simulink model "PSO_ZVD"  (R2021a)
settings: Solver=VariableStepAuto  StartTime=0.0  StopTime=20  RelTol=1e-3
InitFcn:
  | ml=2;
  | 
  | mc=0.5;
  | M2=0.5;
  | 
  | mt=5;
  | g=9.81;
  | l_ref=0.1;
  | l_ini=1;
  | l=l_ini;
  | x_ref=1;
  | n1=5;n2=1;
  | 
  | %ADRC' s parameter caculation
  | %b0 = (ml+mc)/(mc*ml +mc*mt+ml*mt); %Hieu
  | b0=(ml+mc)/(mt*mc+2*ml*mc+mt*ml+ml^2+mc^2); %Enhanced-coupling
  | k_ESO = 100;
  | T_set  = 6;
  | 
  | s_cl = -5.85/T_set;
  | Kp   = s_cl^2;
  | Kd   = -2*s_cl;
  | 
  | s_ESO = k_ESO*s_cl;
  | l1        = -3*s_ESO;
  | l2        = 3*( s_ESO)^2;
  | l3        = -(s_ESO)^3;
  | 
  | %b1 = (mt+mc)/(mc*ml +mc*mt+ml*mt);
  | b1=1/(ml+mc);
  | k_ESO1 =100;
  | T_set1  = 3;
  | s_cl1 = -5.85/T_set1;
  | Kp1   = s_cl1^2;
  | Kd1   = -2*s_cl1;
  | 
  | s_ESO1 = k_ESO1*s_cl1;
  | l11        = -3*s_ESO1;
  | l21        = 3*( s_ESO1)^2;
  | l31        = -(s_ESO1)^3;
  | 
  | 
  | L1=l_ini;
  | %L2=0.5;
  | L2=0.1;
  | m1=2;
  | m2=mc;
  | m=5;
  | %Bo input shaping
  | alpha = (1/L1 + 1/L2)*(m1+M2)/m1;
  | beta = (((m1+M2)/m1)^2)*((1/L1 + 1/L2)^2) - 4*(m1+M2)/(m1*L1*L2);
  | w1 = sqrt(g*(alpha - sqrt(beta))/2);
  | w2 = sqrt(g*(alpha + sqrt(beta))/2);
  | damping_ratio = 0;
  | wd1 = w1*sqrt(1-damping_ratio^2);
  | wd2 = w2*sqrt(1-damping_ratio^2);
  | k = exp(damping_ratio*pi/sqrt(1-damping_ratio^2));
  | 
  | %ZVD1
  | t1_ZVD_1=pi/wd1;
  | t2_ZVD_1=2*pi/wd1;
  | 
  | %ETM4_1
  | m_etm4_1 = 0.1;
  | I_etm4_1 = (1+m_etm4_1)*k*k/(k^2 + (1+m_etm4_1)*(k^(4/3)+k^(2/3)) + m_etm4_1);
  | A1_etm4_1 = I_etm4_1/(1+m_etm4_1);
  | A2_etm4_1 = I_etm4_1/(k^(2/3));
  | A3_etm4_1 = I_etm4_1/(k^(4/3));
  | A4_etm4_1 = m_etm4_1*I_etm4_1/((1+m_etm4_1)*(k^2));
  | t1_etm4_1 = (2*pi/3)/wd1;
  | t2_etm4_1 = (4*pi/3)/wd1;
  | t3_etm4_1 = 2*pi/wd1;
  | 
  | %ZVD1
  | t1_ZVD_2=pi/wd2;
  | t2_ZVD_2=2*pi/wd2;
  | 
  | %ETM4_2
  | m_etm4_2 = 0.1;
  | I_etm4_2 = (1+m_etm4_2)*k*k/(k^2 + (1+m_etm4_2)*(k^(4/3)+k^(2/3)) + m_etm4_2);
  | A1_etm4_2 = I_etm4_2/(1+m_etm4_2);
  | A2_etm4_2 = I_etm4_2/(k^(2/3));
  | A3_etm4_2 = I_etm4_2/(k^(4/3));
  | A4_etm4_2 = m_etm4_2*I_etm4_2/((1+m_etm4_2)*(k^2));
  | t1_etm4_2 = (2*pi/3)/wd2;
  | t2_etm4_2 = (4*pi/3)/wd2;
  | t3_etm4_2 = 2*pi/wd2;
values from neighbouring files (symbols this model uses):
  particle = repmat(empty_particle, nPop, 1)    [PSO16_12.m]    (also in PSO_ZVD.m)
undefined symbols (not defined in the file or in its folder): i, li, xi
libraries: neural x101, simulink_extras x13, simulink x3
(part 1 of 34)
settings Model: Creator=Dao Hieu  LastModifiedBy=Admin

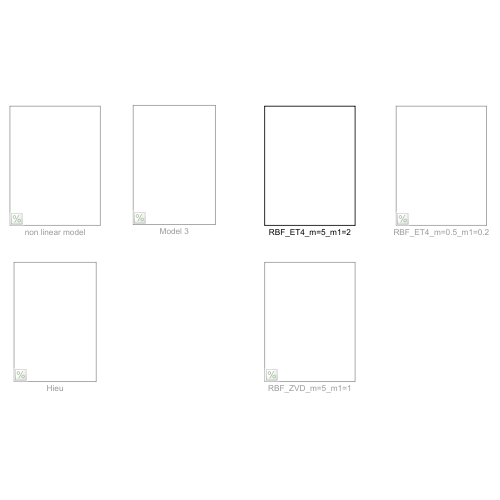
[thumbnail: Simulink's stored preview of the top-level diagram]
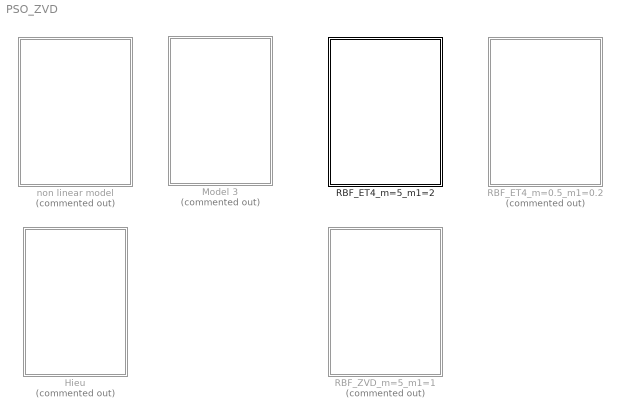
== system PSO_ZVD ==
  Hieu : Subsystem  Commented=on
  Model 3 : Subsystem  Commented=on
  RBF_ET4_m=0.5_m1=0.2 : Subsystem  Commented=on
  RBF_ET4_m=5_m1=2 : Subsystem
  RBF_ZVD_m=5_m1=1 : Subsystem  Commented=on
  non linear model : Subsystem  Commented=on

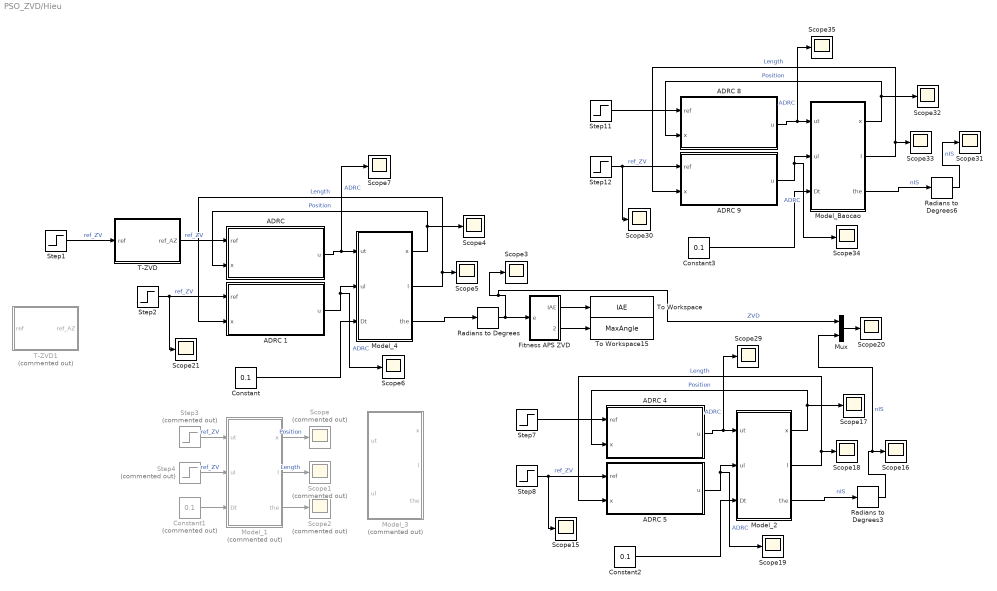
== system PSO_ZVD/Hieu ==
  "ADRC " : Subsystem
  ADRC 1 : Subsystem
  ADRC 4 : Subsystem
  ADRC 5 : Subsystem
  ADRC 8 : Subsystem
  ADRC 9 : Subsystem
  Constant : Constant  Value=0.1
  Constant1 : Constant  Commented=on  Value=0.1
  Constant2 : Constant  Value=0.1
  Constant3 : Constant  Value=0.1
  Fitness APS ZVD : Subsystem
  Model_1 : Subsystem  Commented=on
  Model_2 : Subsystem
  Model_3 : Subsystem  Commented=on
  Model_4 : Subsystem
  Model_Baocao : Subsystem
  Mux : Mux  Inputs=2
  Radians to Degrees : simulink_extras/Transformations/Radians to Degrees
  Radians to Degrees3 : simulink_extras/Transformations/Radians to Degrees
  Radians to Degrees6 : simulink_extras/Transformations/Radians to Degrees
  Scope : Scope  Commented=on
  Scope1 : Scope  Commented=on
  Scope{3..7,15..21,29..35} (19 alike) : Scope
  Scope2 : Scope  Commented=on
  Step1 : Step  SampleTime=0
  Step11 : Step  SampleTime=0
  Step12 : Step  Before=l_ini  After=l_ref  SampleTime=0
  Step2 : Step  Before=l_ini  After=l_ref  SampleTime=0
  Step3 : Step  Commented=on  SampleTime=0
  Step4 : Step  Commented=on  Before=l  After=l  SampleTime=0
  Step7 : Step  SampleTime=0
  Step8 : Step  Before=l_ini  After=l_ref  SampleTime=0
  T-ZVD : Subsystem
  T-ZVD1 : Subsystem  Commented=on
  To Workspace : ToWorkspace  VariableName=IAE  SampleTime=-1
  To Workspace15 : ToWorkspace  VariableName=MaxAngle  SampleTime=-1
  wires:
  Model_1/1(x) -> Scope/1  "Position"
  Fitness APS ZVD/1(IAE) -> To Workspace/1
  Model_4/2(l) -> Scope5/1, ADRC 1/2(x)  "Length"
  Model_Baocao/2(l) -> Scope33/1, ADRC 9/2(x)  "Length"
  Constant1/1 -> Model_1/3(Dt)
  Model_4/1(x) -> Scope4/1, "ADRC "/2(x)  "Position"
  Step8/1 -> ADRC 5/1(ref), Scope15/1  "ref_ZV"
  ADRC 1/1(u) -> Scope6/1, Model_4/2(ul)  "ADRC"
  Model_1/3(the) -> Scope2/1
  Step2/1 -> Scope21/1, ADRC 1/1(ref)  "ref_ZV"
  T-ZVD/1(ref_AZ) -> "ADRC "/1(ref)  "ref_ZV"
  Constant/1 -> Model_4/3(Dt)
  Step7/1 -> ADRC 4/1(ref)
  Step1/1 -> T-ZVD/1(ref)  "ref_ZV"
  Fitness APS ZVD/2(MAx) -> To Workspace15/1
  "ADRC "/1(u) -> Scope7/1, Model_4/1(ut)  "ADRC"
  ADRC 8/1(u) -> Scope35/1, Model_Baocao/1(ut)  "ADRC"
  Radians to Degrees/1 -> Mux/1, Scope3/1, Fitness APS ZVD/1(e)  "ZVD"
  ADRC 4/1(u) -> Scope29/1, Model_2/1(ut)  "ADRC"
  Step12/1 -> Scope30/1, ADRC 9/1(ref)  "ref_ZV"
  Constant2/1 -> Model_2/3(Dt)
  Model_4/3(the) -> Radians to Degrees/1
  Model_Baocao/1(x) -> Scope32/1, ADRC 8/2(x)  "Position"
  Step3/1 -> Model_1/1(ut)  "ref_ZV"
  Model_1/2(l) -> Scope1/1  "Length"
  ADRC 5/1(u) -> Scope19/1, Model_2/2(ul)  "ADRC"
  Constant3/1 -> Model_Baocao/3(Dt)
  Radians to Degrees3/1 -> Mux/2, Scope16/1  "nIS"
  Step11/1 -> ADRC 8/1(ref)
  ADRC 9/1(u) -> Scope34/1, Model_Baocao/2(ul)  "ADRC"
  Model_2/2(l) -> ADRC 5/2(x), Scope18/1  "Length"
  Radians to Degrees6/1 -> Scope31/1  "nIS"
  Mux/1 -> Scope20/1
  Step4/1 -> Model_1/2(ul)  "ref_ZV"
  Model_2/1(x) -> ADRC 4/2(x), Scope17/1  "Position"
  Model_2/3(the) -> Radians to Degrees3/1  "nIS"
  Model_Baocao/3(the) -> Radians to Degrees6/1  "nIS"

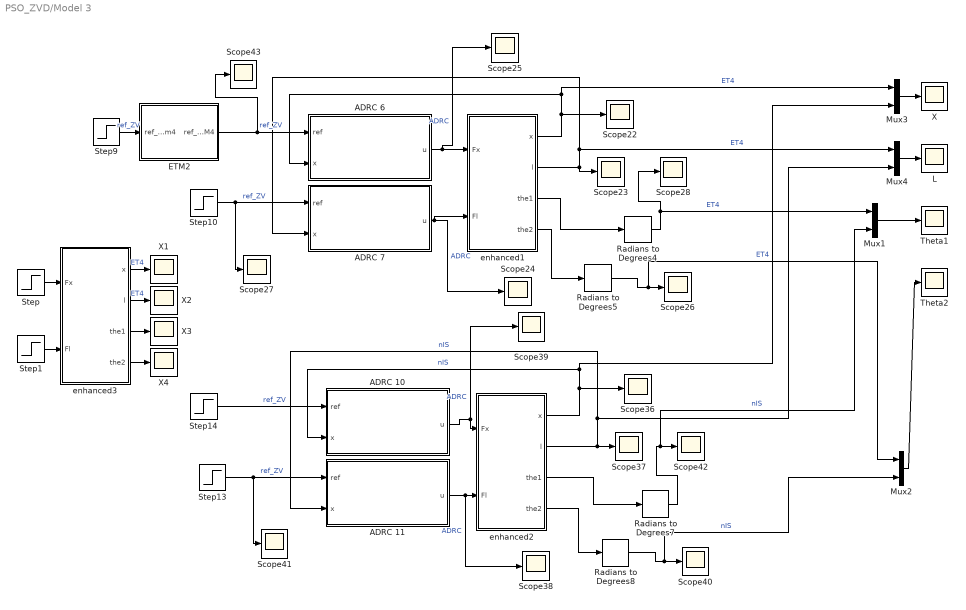
== system PSO_ZVD/Model 3 ==
  ADRC 10 : Subsystem
  ADRC 11 : Subsystem
  ADRC 6 : Subsystem
  ADRC 7 : Subsystem
  ETM2 : Subsystem
  L : Scope
  Mux{1..4} (4 alike) : Mux  Inputs=2
  Radians to Degrees{4..5,7..8} (4 alike) : simulink_extras/Transformations/Radians to Degrees
  Scope{22..28,36..43} (15 alike) : Scope
  Step : Step  Time=0  After=0  SampleTime=0
  Step1 : Step  Time=0  SampleTime=0
  Step10 : Step  Time=0  Before=l_ini  After=l_ref  SampleTime=0
  Step13 : Step  Time=0  Before=l_ini  After=l_ref  SampleTime=0
  Step14 : Step  Time=0  After=x_ref  SampleTime=0
  Step9 : Step  Time=0  After=x_ref  SampleTime=0
  Theta1 : Scope
  Theta2 : Scope
  X{,1..4} (5 alike) : Scope
  enhanced1 : Subsystem
  enhanced2 : Subsystem
  enhanced3 : Subsystem
  wires:
  Radians to Degrees4/1 -> Mux1/1, Scope28/1  "ET4"
  enhanced1/3(the1) -> Radians to Degrees4/1
  ADRC 6/1(u) -> enhanced1/1(Fx), Scope25/1  "ADRC"
  Radians to Degrees7/1 -> Mux1/2, Scope42/1  "nIS"
  Step13/1 -> Scope41/1, ADRC 11/1(ref)  "ref_ZV"
  Radians to Degrees5/1 -> Mux2/1, Scope26/1  "ET4"
  ADRC 11/1(u) -> enhanced2/2(Fl), Scope38/1  "ADRC"
  ADRC 7/1(u) -> enhanced1/2(Fl), Scope24/1  "ADRC"
  ETM2/1(ref_ETM4) -> Scope43/1, ADRC 6/1(ref)  "ref_ZV"
  enhanced2/1(x) -> Scope36/1, Mux3/2, ADRC 10/2(x)  "nIS"
  Step9/1 -> ETM2/1(ref_ETm4)  "ref_ZV"
  Mux1/1 -> Theta1/1
  Step14/1 -> ADRC 10/1(ref)  "ref_ZV"
  Mux2/1 -> Theta2/1
  enhanced1/4(the2) -> Radians to Degrees5/1
  enhanced2/3(the1) -> Radians to Degrees7/1
  Step10/1 -> Scope27/1, ADRC 7/1(ref)  "ref_ZV"
  ADRC 10/1(u) -> enhanced2/1(Fx), Scope39/1  "ADRC"
  Radians to Degrees8/1 -> Mux2/2, Scope40/1  "nIS"
  enhanced2/4(the2) -> Radians to Degrees8/1
  Mux3/1 -> X/1
  enhanced1/1(x) -> Scope22/1, Mux3/1, ADRC 6/2(x)  "ET4"
  enhanced2/2(l) -> Scope37/1, Mux4/2, ADRC 11/2(x)  "nIS"
  enhanced1/2(l) -> Scope23/1, ADRC 7/2(x), Mux4/1  "ET4"
  Mux4/1 -> L/1
  enhanced3/1(x) -> X1/1  "ET4"
  enhanced3/2(l) -> X2/1  "ET4"
  enhanced3/3(the1) -> X3/1
  enhanced3/4(the2) -> X4/1
  Step/1 -> enhanced3/1(Fx)
  Step1/1 -> enhanced3/2(Fl)

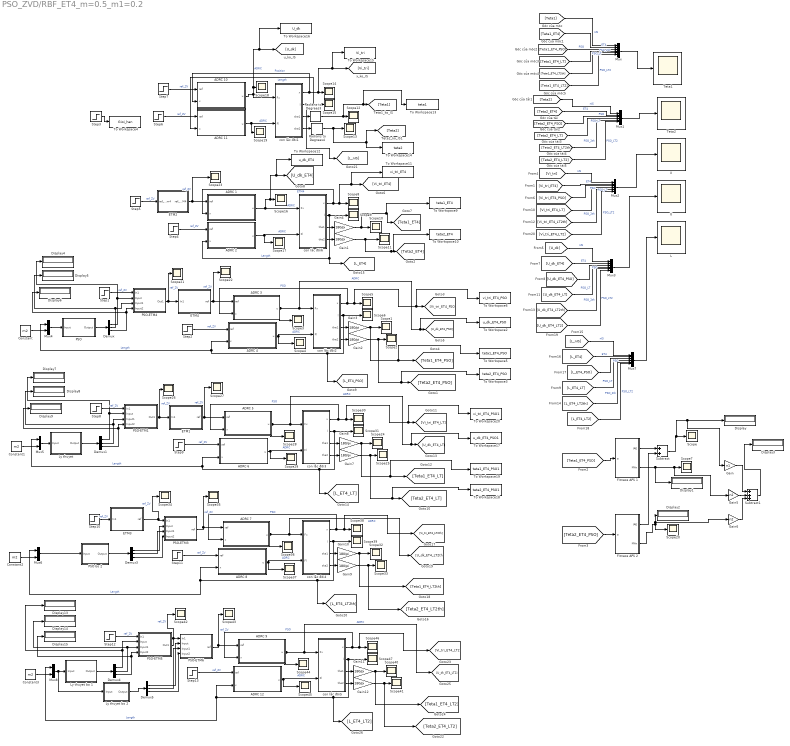
== system PSO_ZVD/RBF_ET4_m=0.5_m1=0.2 ==
  ADRC 1 : Subsystem
  ADRC 10 : Subsystem
  ADRC 11 : Subsystem
  ADRC 12 : Subsystem
  ADRC 2 : Subsystem
  ADRC 3 : Subsystem
  ADRC 4 : Subsystem
  ADRC 5 : Subsystem
  ADRC 6 : Subsystem
  ADRC 7 : Subsystem
  ADRC 8 : Subsystem
  ADRC 9 : Subsystem
  Constant{,1..3} (4 alike) : Constant  Value=m2
  Demux{,1,3..5} (5 alike) : Demux  Outputs=3
  Display{,1..9,13..15} (13 alike) : Display
  ETM1 : Subsystem
  ETM2 : Subsystem
  ETM3 : Subsystem
  ETM4 : Subsystem
  Fitness APS 1 : Subsystem
  Fitness APS 2 : Subsystem
  Gain : Gain  Gain=n1
  Gain{1..4,7..12} (10 alike) : Gain  Gain=180/pi
  Gain5 : Gain  Gain=n2
  Gain6 : Gain  Gain=n2
  L : Scope
  Ly thuyet : Subsystem
      mask help: Radial Basis Network
      mask Display: e = 0.06;c1 = [120 150 230]/255;c2 = ([120 150 230]+0)/383;c3 = ([120 150 230]+128)/383;patch([0 1 1 0],[0 0 1 1],c1);patch([0 1 1 1-e 1-e 0+e],[0 0 1 1-e 0+e 0+e],c2);patch([0 0 1 1-e 0+e 0+e],[0 1 1 1-e 1-e 0+e],c3);plot([0 1 1 0 0],[0 0 1 1 0]);fprintf('NNET');port_label('input',1,' Input');port_label('output',1,'Output ');
  Ly thuyet bo 1 : Subsystem
      mask help: Radial Basis Network
      mask Display: e = 0.06;c1 = [120 150 230]/255;c2 = ([120 150 230]+0)/383;c3 = ([120 150 230]+128)/383;patch([0 1 1 0],[0 0 1 1],c1);patch([0 1 1 1-e 1-e 0+e],[0 0 1 1-e 0+e 0+e],c2);patch([0 0 1 1-e 0+e 0+e],[0 1 1 1-e 1-e 0+e],c3);plot([0 1 1 0 0],[0 0 1 1 0]);fprintf('NNET');port_label('input',1,' Input');port_label('output',1,'Output ');
  Ly thuyet bo 2 : Subsystem
      mask help: Radial Basis Network
      mask Display: e = 0.06;c1 = [120 150 230]/255;c2 = ([120 150 230]+0)/383;c3 = ([120 150 230]+128)/383;patch([0 1 1 0],[0 0 1 1],c1);patch([0 1 1 1-e 1-e 0+e],[0 0 1 1-e 0+e 0+e],c2);patch([0 0 1 1-e 0+e 0+e],[0 1 1 1-e 1-e 0+e],c3);plot([0 1 1 0 0],[0 0 1 1 0]);fprintf('NNET');port_label('input',1,' Input');port_label('output',1,'Output ');
  Mux{,1..3,7} (5 alike) : Mux  Inputs=6
  Mux{4..6,8} (4 alike) : Mux  Inputs=2
  PSO : Subsystem
      mask help: Radial Basis Network
      mask Display: e = 0.06;c1 = [120 150 230]/255;c2 = ([120 150 230]+0)/383;c3 = ([120 150 230]+128)/383;patch([0 1 1 0],[0 0 1 1],c1);patch([0 1 1 1-e 1-e 0+e],[0 0 1 1-e 0+e 0+e],c2);patch([0 0 1 1-e 0+e 0+e],[0 1 1 1-e 1-e 0+e],c3);plot([0 1 1 0 0],[0 0 1 1 0]);fprintf('NNET');port_label('input',1,' Input');port_label('output',1,'Output ');
  PSO bo 2 : Subsystem
      mask help: Radial Basis Network
      mask Display: e = 0.06;c1 = [120 150 230]/255;c2 = ([120 150 230]+0)/383;c3 = ([120 150 230]+128)/383;patch([0 1 1 0],[0 0 1 1],c1);patch([0 1 1 1-e 1-e 0+e],[0 0 1 1-e 0+e 0+e],c2);patch([0 0 1 1-e 0+e 0+e],[0 1 1 1-e 1-e 0+e],c3);plot([0 1 1 0 0],[0 0 1 1 0]);fprintf('NNET');port_label('input',1,' Input');port_label('output',1,'Output ');
  PSO-ETM1 : Subsystem
  PSO-ETM3 : Subsystem
  PSO-ETM4 : Subsystem
  PSO-ETM5 : Subsystem
  PSO-ETM6 : Subsystem
  Radians to Degrees3 : simulink_extras/Transformations/Radians to Degrees
  Radians to Degrees4 : simulink_extras/Transformations/Radians to Degrees
  Scope{,1..47} (48 alike) : Scope
  Step{1,5,7..8,10,12} (6 alike) : Step  Time=0  After=x_ref  SampleTime=0
  Step{2,4,6,9,11,13} (6 alike) : Step  Time=0  Before=l_ini  After=l_ref  SampleTime=0
  Step3 : Step  Time=0  After=10  SampleTime=0
  Subtract : Sum
  Subtract1 : Sum  Inputs=+++
  Teta1 : Scope
  Teta2 : Scope
  To Workspace10 : ToWorkspace  VariableName=teta2_ET4  SaveFormat=Timeseries  SampleTime=-1
  To Workspace11 : ToWorkspace  VariableName=vi_tri_ET4  SaveFormat=Timeseries  SampleTime=-1
  To Workspace12 : ToWorkspace  VariableName=u_dk_ET4  SaveFormat=Timeseries  SampleTime=-1
  To Workspace13 : ToWorkspace  VariableName=teta1  SaveFormat=Timeseries  SampleTime=-1
  To Workspace14 : ToWorkspace  VariableName=teta2  SaveFormat=Timeseries  SampleTime=-1
  To Workspace15 : ToWorkspace  VariableName=Vi_tri  SaveFormat=Timeseries  SampleTime=-1
  To Workspace16 : ToWorkspace  VariableName=U_dk  SaveFormat=Timeseries  SampleTime=-1
  To Workspace17 : ToWorkspace  VariableName=u_dk_ET4_PSO1  SaveFormat=Timeseries  SampleTime=-1
  To Workspace18 : ToWorkspace  VariableName=teta2_ET4_PSO1  SaveFormat=Timeseries  SampleTime=-1
  To Workspace19 : ToWorkspace  VariableName=teta1_ET4_PSO1  SaveFormat=Timeseries  SampleTime=-1
  To Workspace2 : ToWorkspace  VariableName=u_dk_ET4_PSO  SaveFormat=Timeseries  SampleTime=-1
  To Workspace20 : ToWorkspace  VariableName=vi_tri_ET4_PSO1  SaveFormat=Timeseries  SampleTime=-1
  To Workspace3 : ToWorkspace  VariableName=teta2_ET4_PSO  SaveFormat=Timeseries  SampleTime=-1
  To Workspace4 : ToWorkspace  VariableName=Gioi_han  SaveFormat=Timeseries  SampleTime=-1
  To Workspace5 : ToWorkspace  VariableName=teta1_ET4_PSO  SaveFormat=Timeseries  SampleTime=-1
  To Workspace6 : ToWorkspace  VariableName=vi_tri_ET4_PSO  SaveFormat=Timeseries  SampleTime=-1
  To Workspace9 : ToWorkspace  VariableName=teta1_ET4  SaveFormat=Timeseries  SampleTime=-1
  U : Scope
  X : Scope
  con lắc đôi1 : Subsystem
  con lắc đôi2 : Subsystem
  con lắc đôi3 : Subsystem
  con lắc đôi4 : Subsystem
  con lắc đôi5 : Subsystem
  con lắc đôi6 : Subsystem
  wires:
  ADRC 2/1(u) -> con lắc đôi6/2(Fl), Scope17/1  "ADRC"
  ADRC 11/1(u) -> con lắc đôi1/2(Fl), Scope19/1  "ADRC"
  ADRC 1/1(u) -> con lắc đôi6/1(Fx), To Workspace12/1, [U_dk_ET4], Scope16/1  "ADRC"
  con lắc đôi6/1(x) -> ADRC 1/2(x), To Workspace11/1, [Vi_tri_ET4], Scope8/1  "ETM4"
  con lắc đôi1/3(the1) -> Radians to Degrees3/1
  con lắc đôi6/2(l) -> [L_ET4], ADRC 2/2(x), Scope9/1  "Length"
  con lắc đôi1/1(x) -> ADRC 10/2(x), To Workspace15/1, [Vi_tri], Scope14/1  "Position"
  Step6/1 -> ADRC 11/1(ref)  "ref_ZV"
  Step4/1 -> ADRC 2/1(ref)  "ref_ZV"
  con lắc đôi1/2(l) -> Scope15/1, ADRC 11/2(x), [L_nIS]  "Length"
  Step7/1 -> ADRC 10/1(ref)  "ref_ZV"
  Gain4/1 -> To Workspace9/1, [Teta1_ET4], Scope10/1
  ETM2/1(ref_ETM4) -> ADRC 1/1(ref), Scope23/1  "ref_ZV"
  Step5/1 -> ETM2/1(ref_ETm4)  "ref_ZV"
  ADRC 10/1(u) -> con lắc đôi1/1(Fx), To Workspace16/1, [U_dk], Scope18/1  "ADRC"
  Radians to Degrees3/1 -> To Workspace13/1, [Teta1], Scope12/1
  con lắc đôi1/4(the2) -> Radians to Degrees4/1
  con lắc đôi6/3(the1) -> Gain4/1
  Gain1/1 -> To Workspace10/1, [Teta2_ET4], Scope11/1
  con lắc đôi6/4(the2) -> Gain1/1
  Radians to Degrees4/1 -> [Teta2], To Workspace14/1, Scope13/1
  ADRC 4/1(u) -> con lắc đôi2/2(Fl), Scope4/1  "ADRC"
  con lắc đôi2/4(the2) -> Gain2/1
  Step1/1 -> PSO-ETM4/1(In1)  "ref_ZV"
  ADRC 3/1(u) -> Scope3/1, con lắc đôi2/1(Fx), To Workspace2/1, [U_dk_ET4_PSO]  "ADRC"
  con lắc đôi2/1(x) -> ADRC 3/2(x), To Workspace6/1, [Vi_tri_ET4_PSO], Scope5/1  "PSO"
  con lắc đôi2/2(l) -> Scope6/1, [L_ET4_PSO], ADRC 4/2(x), Mux4/1  "Length"
  Gain3/1 -> [Teta1_ET4_PSO], To Workspace5/1, Scope1/1
  Step2/1 -> ADRC 4/1(ref)  "ref_ZV"
  con lắc đôi2/3(the1) -> Gain3/1
  PSO-ETM4/1(Out1) -> Scope21/1, ETM4/1(In1)  "ref_ZV"
  [Teta2] -> Mux1/1  "nIS"
  Subtract/1 -> Gain/1, Display/1, Scope/1
  [U_dk] -> Mux3/1  "nIS"
  [U_dk_ET4] -> Mux3/2  "ET4"
  [Teta2_ET4_PSO] -> Fitness APS 2/1(e)
  [Teta1_ET4_PSO] -> Fitness APS 1/1(e)
  [Vi_tri] -> Mux2/1  "nIS"
  [Teta2_ET4] -> Mux1/2  "ET4"
  [Vi_tri_ET4] -> Mux2/2  "ET4"
  [Teta1] -> Mux/1  "nIS"
  Gain5/1 -> Subtract1/2
  Fitness APS 2/2(MAx) -> Gain6/1, Display2/1, Scope20/1
  Mux2/1 -> X/1
  Gain6/1 -> Subtract1/3
  Mux/1 -> Teta1/1
  Mux1/1 -> Teta2/1
  Mux3/1 -> U/1
  Gain/1 -> Subtract1/1
  [Teta1_ET4] -> Mux/2  "ET4"
  Fitness APS 2/1(IAE) -> Subtract/2
  Subtract1/1 -> Display3/1
  Fitness APS 1/1(IAE) -> Subtract/1
  Fitness APS 1/2(MAx) -> Display1/1, Gain5/1, Scope7/1
  Step3/1 -> To Workspace4/1
  Gain2/1 -> [Teta2_ET4_PSO], To Workspace3/1, Scope2/1
  [Teta2_ET4_PSO] -> Mux1/3  "PSO"
  [Vi_tri_ET4_PSO] -> Mux2/3  "PSO"
  [Teta1_ET4_PSO] -> Mux/3  "PSO"
  [U_dk_ET4_PSO] -> Mux3/3  "PSO"
  Constant/1 -> Mux4/2
  Mux4/1 -> PSO/1(Input)
  Demux/1 -> PSO-ETM4/2(Input), Display4/1
  Demux/2 -> Display5/1, PSO-ETM4/3(Input1)
  Demux/3 -> Display6/1, PSO-ETM4/4(Input2)
  ETM4/1(ref) -> ADRC 3/1(ref), Scope22/1  "ref_ZV"
  PSO/1(Output) -> Demux/1
  Demux1/1 -> PSO-ETM1/2(Input), Display7/1
  Mux5/1 -> Ly thuyet/1(Input)
  Constant1/1 -> Mux5/2
  con lắc đôi3/1(x) -> ADRC 5/2(x), To Workspace20/1, [Vi_tri_ET4_LT], Scope30/1  "PSO"
  Gain7/1 -> [Teta2_ET4_LT], To Workspace18/1, Scope25/1
  con lắc đôi3/3(the1) -> Gain8/1
  Step9/1 -> ADRC 6/1(ref)  "ref_ZV"
  ETM1/1(ref) -> ADRC 5/1(ref), Scope27/1  "ref_ZV"
  PSO-ETM1/1(Out1) -> Scope26/1, ETM1/1(In1)  "ref_ZV"
  ADRC 5/1(u) -> Scope28/1, con lắc đôi3/1(Fx), To Workspace17/1, [U_dk_ET4_LT]  "ADRC"
  Demux1/2 -> Display8/1, PSO-ETM1/3(Input1)
  Demux1/3 -> Display9/1, PSO-ETM1/4(Input2)
  ADRC 6/1(u) -> con lắc đôi3/2(Fl), Scope29/1  "ADRC"
  con lắc đôi3/2(l) -> Scope31/1, [L_ET4_LT], ADRC 6/2(x), Mux5/1  "Length"
  Ly thuyet/1(Output) -> Demux1/1
  Gain8/1 -> [Teta1_ET4_LT], To Workspace19/1, Scope24/1
  con lắc đôi3/4(the2) -> Gain7/1
  Step8/1 -> PSO-ETM1/1(In1)  "ref_ZV"
  [Teta1_ET4_LT] -> Mux/4  "PSO_LT"
  [Teta2_ET4_LT] -> Mux1/4  "PSO_LT"
  [Vi_tri_ET4_LT] -> Mux2/4  "PSO_LT"
  [U_dk_ET4_LT] -> Mux3/4  "PSO_LT"
  PSO-ETM3/1(ref) -> ADRC 7/1(ref), Scope35/1  "ref_ZV"
  Step11/1 -> ADRC 8/1(ref)  "ref_ZV"
  Demux3/1 -> PSO-ETM3/2(Input)
  Demux3/2 -> PSO-ETM3/3(Input1)
  ETM3/1(ref) -> PSO-ETM3/1(In1), Scope34/1  "ref_ZV"
  con lắc đôi4/2(l) -> Scope39/1, [L_ET4_LT2th], ADRC 8/2(x), Mux6/1  "Length"
  Gain10/1 -> [Teta1_ET4_LT2th], Scope32/1
  ADRC 8/1(u) -> con lắc đôi4/2(Fl), Scope37/1  "ADRC"
  con lắc đôi4/1(x) -> ADRC 7/2(x), [Vi_tri_ET4_LT2th], Scope38/1  "PSO"
  Step10/1 -> ETM3/1(In1)  "ref_ZV"
  Constant2/1 -> Mux6/2
  ADRC 7/1(u) -> Scope36/1, con lắc đôi4/1(Fx), [U_dk_ET4_LT2th]  "ADRC"
  con lắc đôi4/4(the2) -> Gain9/1
  Mux6/1 -> PSO bo 2/1(Input)
  con lắc đôi4/3(the1) -> Gain10/1
  PSO bo 2/1(Output) -> Demux3/1
  Demux3/3 -> PSO-ETM3/4(Input2)
  Gain9/1 -> [Teta2_ET4_LT2th], Scope33/1
  [Teta1_ET4_LT2th] -> Mux/5  "PSO_2th"
  [Teta2_ET4_LT2th] -> Mux1/5  "PSO_2th"
  [Vi_tri_ET4_LT2th] -> Mux2/5  "PSO_2th"
  [U_dk_ET4_LT2th] -> Mux3/5  "PSO_2th"
  [L_ET4] -> Mux7/2  "ET4"
  [L_nIS] -> Mux7/1  "nIS"
  [L_ET4_LT2th] -> Mux7/5  "PSO_2th"
  [L_ET4_LT] -> Mux7/4  "PSO_LT"
  Mux7/1 -> L/1
  [L_ET4_PSO] -> Mux7/3  "PSO"
  con lắc đôi5/3(the1) -> Gain11/1
  con lắc đôi5/1(x) -> ADRC 9/2(x), [Vi_tri_ET4_LT2], Scope46/1  "PSO"
  ADRC 9/1(u) -> Scope44/1, con lắc đôi5/1(Fx), [U_dk_ET4_LT2]  "ADRC"
  Gain12/1 -> [Teta2_ET4_LT2], Scope41/1
  Ly thuyet bo 1/1(Output) -> Demux4/1
  ADRC 12/1(u) -> con lắc đôi5/2(Fl), Scope45/1  "ADRC"
  Demux4/3 -> Display15/1, PSO-ETM5/4(Input2)
  PSO-ETM6/1(ref) -> ADRC 9/1(ref), Scope43/1  "ref_ZV"
  con lắc đôi5/4(the2) -> Gain12/1
  Step12/1 -> PSO-ETM5/1(In1)  "ref_ZV"
  Demux5/2 -> PSO-ETM6/3(Input1)
  Demux4/2 -> Display14/1, PSO-ETM5/3(Input1)
  Constant3/1 -> Mux8/2
  Gain11/1 -> [Teta1_ET4_LT2], Scope40/1
  Demux5/3 -> PSO-ETM6/4(Input2)
  con lắc đôi5/2(l) -> Scope47/1, [L_ET4_LT2], ADRC 12/2(x), Mux8/1  "Length"
  Ly thuyet bo 2/1(Output) -> Demux5/1
  PSO-ETM5/1(Out1) -> PSO-ETM6/1(In1), Scope42/1  "ref_ZV"
  Demux4/1 -> PSO-ETM5/2(Input), Display13/1
  Mux8/1 -> Ly thuyet bo 2/1(Input), Ly thuyet bo 1/1(Input)
  Demux5/1 -> PSO-ETM6/2(Input)
  Step13/1 -> ADRC 12/1(ref)  "ref_ZV"
  [Teta1_ET4_LT2] -> Mux/6  "PSO_LT2"
  [Teta2_ET4_LT2] -> Mux1/6  "PSO_LT2"
  [L_ET4_LT2] -> Mux7/6  "PSO_LT2"
  [U_dk_ET4_LT2] -> Mux3/6  "PSO_LT2"
  [Vi_tri_ET4_LT2] -> Mux2/6  "PSO_LT2"

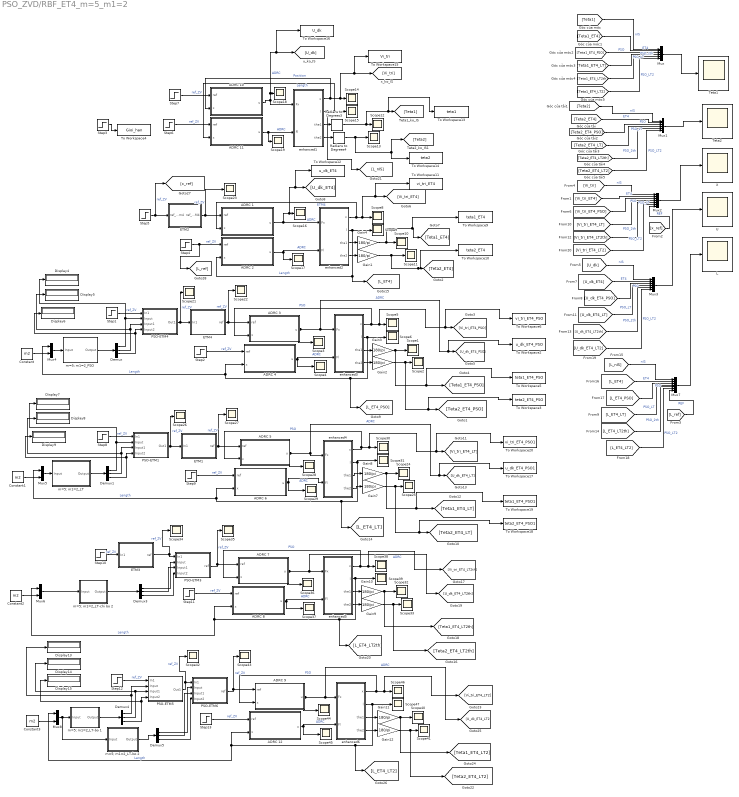
== system PSO_ZVD/RBF_ET4_m=5_m1=2 ==
  ADRC 1 : Subsystem
  ADRC 10 : Subsystem
  ADRC 11 : Subsystem
  ADRC 12 : Subsystem
  ADRC 2 : Subsystem
  ADRC 3 : Subsystem
  ADRC 4 : Subsystem
  ADRC 5 : Subsystem
  ADRC 6 : Subsystem
  ADRC 7 : Subsystem
  ADRC 8 : Subsystem
  ADRC 9 : Subsystem
  Constant{,1..3} (4 alike) : Constant  Value=m2
  Demux{,1,3..5} (5 alike) : Demux  Outputs=3
  Display{4..9,13..15} (9 alike) : Display
  ETM1 : Subsystem
  ETM2 : Subsystem
  ETM3 : Subsystem
  ETM4 : Subsystem
  Gain{1..4,7..12} (10 alike) : Gain  Gain=180/pi
  L : Scope
  Mux : Mux  Inputs=6
  Mux1 : Mux  Inputs=6
  Mux2 : Mux  Inputs=7
  Mux3 : Mux  Inputs=6
  Mux{4..6,8} (4 alike) : Mux  Inputs=2
  Mux7 : Mux  Inputs=7
  PSO-ETM1 : Subsystem
  PSO-ETM3 : Subsystem
  PSO-ETM4 : Subsystem
  PSO-ETM5 : Subsystem
  PSO-ETM6 : Subsystem
  Radians to Degrees3 : simulink_extras/Transformations/Radians to Degrees
  Radians to Degrees4 : simulink_extras/Transformations/Radians to Degrees
  Scope{1..6,8..19,21..47} (45 alike) : Scope
  Step{1,5,7..8,10,12} (6 alike) : Step  Time=0  After=x_ref  SampleTime=0
  Step{2,4,6,9,11,13} (6 alike) : Step  Time=0  Before=l_ini  After=l_ref  SampleTime=0
  Step3 : Step  Time=0  After=10  SampleTime=0
  Teta1 : Scope
  Teta2 : Scope
  To Workspace10 : ToWorkspace  VariableName=teta2_ET4  SaveFormat=Timeseries  SampleTime=-1
  To Workspace11 : ToWorkspace  VariableName=vi_tri_ET4  SaveFormat=Timeseries  SampleTime=-1
  To Workspace12 : ToWorkspace  VariableName=u_dk_ET4  SaveFormat=Timeseries  SampleTime=-1
  To Workspace13 : ToWorkspace  VariableName=teta1  SaveFormat=Timeseries  SampleTime=-1
  To Workspace14 : ToWorkspace  VariableName=teta2  SaveFormat=Timeseries  SampleTime=-1
  To Workspace15 : ToWorkspace  VariableName=Vi_tri  SaveFormat=Timeseries  SampleTime=-1
  To Workspace16 : ToWorkspace  VariableName=U_dk  SaveFormat=Timeseries  SampleTime=-1
  To Workspace17 : ToWorkspace  VariableName=u_dk_ET4_PSO1  SaveFormat=Timeseries  SampleTime=-1
  To Workspace18 : ToWorkspace  VariableName=teta2_ET4_PSO1  SaveFormat=Timeseries  SampleTime=-1
  To Workspace19 : ToWorkspace  VariableName=teta1_ET4_PSO1  SaveFormat=Timeseries  SampleTime=-1
  To Workspace2 : ToWorkspace  VariableName=u_dk_ET4_PSO  SaveFormat=Timeseries  SampleTime=-1
  To Workspace20 : ToWorkspace  VariableName=vi_tri_ET4_PSO1  SaveFormat=Timeseries  SampleTime=-1
  To Workspace3 : ToWorkspace  VariableName=teta2_ET4_PSO  SaveFormat=Timeseries  SampleTime=-1
  To Workspace4 : ToWorkspace  VariableName=Gioi_han  SaveFormat=Timeseries  SampleTime=-1
  To Workspace5 : ToWorkspace  VariableName=teta1_ET4_PSO  SaveFormat=Timeseries  SampleTime=-1
  To Workspace6 : ToWorkspace  VariableName=vi_tri_ET4_PSO  SaveFormat=Timeseries  SampleTime=-1
  To Workspace9 : ToWorkspace  VariableName=teta1_ET4  SaveFormat=Timeseries  SampleTime=-1
  U : Scope
  X : Scope
  enhanced1 : Subsystem
  enhanced2 : Subsystem
  enhanced3 : Subsystem
  enhanced4 : Subsystem
  enhanced5 : Subsystem
  enhanced6 : Subsystem
  m=5; m1=2_LT : Subsystem
      mask help: Radial Basis Network
      mask Display: e = 0.06;c1 = [120 150 230]/255;c2 = ([120 150 230]+0)/383;c3 = ([120 150 230]+128)/383;patch([0 1 1 0],[0 0 1 1],c1);patch([0 1 1 1-e 1-e 0+e],[0 0 1 1-e 0+e 0+e],c2);patch([0 0 1 1-e 0+e 0+e],[0 1 1 1-e 1-e 0+e],c3);plot([0 1 1 0 0],[0 0 1 1 0]);fprintf('NNET');port_label('input',1,' Input');port_label('output',1,'Output ');
  m=5; m1=2_LT-bo 1 : Subsystem
      mask help: Radial Basis Network
      mask Display: e = 0.06;c1 = [120 150 230]/255;c2 = ([120 150 230]+0)/383;c3 = ([120 150 230]+128)/383;patch([0 1 1 0],[0 0 1 1],c1);patch([0 1 1 1-e 1-e 0+e],[0 0 1 1-e 0+e 0+e],c2);patch([0 0 1 1-e 0+e 0+e],[0 1 1 1-e 1-e 0+e],c3);plot([0 1 1 0 0],[0 0 1 1 0]);fprintf('NNET');port_label('input',1,' Input');port_label('output',1,'Output ');
  m=5; m1=2_LT-bo 2 : Subsystem
      mask help: Radial Basis Network
      mask Display: e = 0.06;c1 = [120 150 230]/255;c2 = ([120 150 230]+0)/383;c3 = ([120 150 230]+128)/383;patch([0 1 1 0],[0 0 1 1],c1);patch([0 1 1 1-e 1-e 0+e],[0 0 1 1-e 0+e 0+e],c2);patch([0 0 1 1-e 0+e 0+e],[0 1 1 1-e 1-e 0+e],c3);plot([0 1 1 0 0],[0 0 1 1 0]);fprintf('NNET');port_label('input',1,' Input');port_label('output',1,'Output ');
  m=5; m1=2_LT-chi bo 2 : Subsystem
      mask help: Radial Basis Network
      mask Display: e = 0.06;c1 = [120 150 230]/255;c2 = ([120 150 230]+0)/383;c3 = ([120 150 230]+128)/383;patch([0 1 1 0],[0 0 1 1],c1);patch([0 1 1 1-e 1-e 0+e],[0 0 1 1-e 0+e 0+e],c2);patch([0 0 1 1-e 0+e 0+e],[0 1 1 1-e 1-e 0+e],c3);plot([0 1 1 0 0],[0 0 1 1 0]);fprintf('NNET');port_label('input',1,' Input');port_label('output',1,'Output ');
  m=5; m1=2_PSO : Subsystem
      mask help: Radial Basis Network
      mask Display: e = 0.06;c1 = [120 150 230]/255;c2 = ([120 150 230]+0)/383;c3 = ([120 150 230]+128)/383;patch([0 1 1 0],[0 0 1 1],c1);patch([0 1 1 1-e 1-e 0+e],[0 0 1 1-e 0+e 0+e],c2);patch([0 0 1 1-e 0+e 0+e],[0 1 1 1-e 1-e 0+e],c3);plot([0 1 1 0 0],[0 0 1 1 0]);fprintf('NNET');port_label('input',1,' Input');port_label('output',1,'Output ');
  wires:
  ADRC 2/1(u) -> enhanced2/2(Fl), Scope17/1  "ADRC"
  ADRC 11/1(u) -> enhanced1/2(Fl), Scope19/1  "ADRC"
  ADRC 1/1(u) -> enhanced2/1(Fx), To Workspace12/1, [U_dk_ET4], Scope16/1  "ADRC"
  enhanced2/1(x) -> ADRC 1/2(x), To Workspace11/1, [Vi_tri_ET4], Scope8/1  "ETM4"
  enhanced1/3(the1) -> Radians to Degrees3/1
  enhanced2/2(l) -> [L_ET4], ADRC 2/2(x), Scope9/1  "Length"
  enhanced1/1(x) -> ADRC 10/2(x), To Workspace15/1, [Vi_tri], Scope14/1  "Position"
  Step6/1 -> ADRC 11/1(ref)  "ref_ZV"
  Step4/1 -> [L_ref], ADRC 2/1(ref)  "ref_ZV"
  enhanced1/2(l) -> Scope15/1, ADRC 11/2(x), [L_nIS]  "Length"
  Step7/1 -> ADRC 10/1(ref)  "ref_ZV"
  Gain4/1 -> To Workspace9/1, [Teta1_ET4], Scope10/1
  ETM2/1(ref_ETM4) -> ADRC 1/1(ref), Scope23/1  "ref_ZV"
  Step5/1 -> [x_ref], ETM2/1(ref_ETm4)  "ref_ZV"
  ADRC 10/1(u) -> enhanced1/1(Fx), To Workspace16/1, [U_dk], Scope18/1  "ADRC"
  Radians to Degrees3/1 -> To Workspace13/1, [Teta1], Scope12/1
  enhanced1/4(the2) -> Radians to Degrees4/1
  enhanced2/3(the1) -> Gain4/1
  Gain1/1 -> To Workspace10/1, [Teta2_ET4], Scope11/1
  enhanced2/4(the2) -> Gain1/1
  Radians to Degrees4/1 -> [Teta2], To Workspace14/1, Scope13/1
  ADRC 4/1(u) -> enhanced3/2(Fl), Scope4/1  "ADRC"
  enhanced3/4(the2) -> Gain2/1
  Step1/1 -> PSO-ETM4/1(In1)  "ref_ZV"
  ADRC 3/1(u) -> Scope3/1, enhanced3/1(Fx), To Workspace2/1, [U_dk_ET4_PSO]  "ADRC"
  enhanced3/1(x) -> ADRC 3/2(x), To Workspace6/1, [Vi_tri_ET4_PSO], Scope5/1  "PSO"
  enhanced3/2(l) -> Scope6/1, [L_ET4_PSO], ADRC 4/2(x), Mux4/1  "Length"
  Gain3/1 -> [Teta1_ET4_PSO], To Workspace5/1, Scope1/1
  Step2/1 -> ADRC 4/1(ref)  "ref_ZV"
  enhanced3/3(the1) -> Gain3/1
  PSO-ETM4/1(Out1) -> Scope21/1, ETM4/1(In1)  "ref_ZV"
  [Teta2] -> Mux1/1  "nIS"
  [U_dk] -> Mux3/1  "nIS"
  [U_dk_ET4] -> Mux3/2  "ET4"
  [Vi_tri] -> Mux2/1  "nIS"
  [Teta2_ET4] -> Mux1/2  "ET4"
  [Vi_tri_ET4] -> Mux2/2  "ET4"
  [Teta1] -> Mux/1  "nIS"
  Mux2/1 -> X/1
  Mux/1 -> Teta1/1
  Mux1/1 -> Teta2/1
  Mux3/1 -> U/1
  [Teta1_ET4] -> Mux/2  "ET4"
  Step3/1 -> To Workspace4/1
  Gain2/1 -> [Teta2_ET4_PSO], To Workspace3/1, Scope2/1
  [Teta2_ET4_PSO] -> Mux1/3  "PSO"
  [Vi_tri_ET4_PSO] -> Mux2/3  "PSO"
  [Teta1_ET4_PSO] -> Mux/3  "PSO"
  [U_dk_ET4_PSO] -> Mux3/3  "PSO"
  Constant/1 -> Mux4/2
  Mux4/1 -> m=5; m1=2_PSO/1(Input)
  Demux/1 -> PSO-ETM4/2(Input), Display4/1
  Demux/2 -> Display5/1, PSO-ETM4/3(Input1)
  Demux/3 -> Display6/1, PSO-ETM4/4(Input2)
  ETM4/1(ref) -> ADRC 3/1(ref), Scope22/1  "ref_ZV"
  m=5; m1=2_PSO/1(Output) -> Demux/1
  Demux1/1 -> PSO-ETM1/2(Input), Display7/1
  Mux5/1 -> m=5; m1=2_LT/1(Input)
  Constant1/1 -> Mux5/2
  enhanced4/1(x) -> ADRC 5/2(x), To Workspace20/1, [Vi_tri_ET4_LT], Scope30/1  "PSO"
  Gain7/1 -> [Teta2_ET4_LT], To Workspace18/1, Scope25/1
  enhanced4/3(the1) -> Gain8/1
  Step9/1 -> ADRC 6/1(ref)  "ref_ZV"
  ETM1/1(ref) -> ADRC 5/1(ref), Scope27/1  "ref_ZV"
  PSO-ETM1/1(Out1) -> Scope26/1, ETM1/1(In1)  "ref_ZV"
  ADRC 5/1(u) -> Scope28/1, enhanced4/1(Fx), To Workspace17/1, [U_dk_ET4_LT]  "ADRC"
  Demux1/2 -> Display8/1, PSO-ETM1/3(Input1)
  Demux1/3 -> Display9/1, PSO-ETM1/4(Input2)
  ADRC 6/1(u) -> enhanced4/2(Fl), Scope29/1  "ADRC"
  enhanced4/2(l) -> Scope31/1, [L_ET4_LT], ADRC 6/2(x), Mux5/1  "Length"
  m=5; m1=2_LT/1(Output) -> Demux1/1
  Gain8/1 -> [Teta1_ET4_LT], To Workspace19/1, Scope24/1
  enhanced4/4(the2) -> Gain7/1
  Step8/1 -> PSO-ETM1/1(In1)  "ref_ZV"
  [Teta1_ET4_LT] -> Mux/4  "PSO_LT"
  [Teta2_ET4_LT] -> Mux1/4  "PSO_LT"
  [Vi_tri_ET4_LT] -> Mux2/4  "PSO_LT"
  [U_dk_ET4_LT] -> Mux3/4  "PSO_LT"
  PSO-ETM3/1(ref) -> ADRC 7/1(ref), Scope35/1  "ref_ZV"
  Step11/1 -> ADRC 8/1(ref)  "ref_ZV"
  Demux3/1 -> PSO-ETM3/2(Input)
  Demux3/2 -> PSO-ETM3/3(Input1)
  ETM3/1(ref) -> PSO-ETM3/1(In1), Scope34/1  "ref_ZV"
  enhanced5/2(l) -> Scope39/1, [L_ET4_LT2th], ADRC 8/2(x), Mux6/1  "Length"
  Gain10/1 -> [Teta1_ET4_LT2th], Scope32/1
  ADRC 8/1(u) -> enhanced5/2(Fl), Scope37/1  "ADRC"
  enhanced5/1(x) -> ADRC 7/2(x), [Vi_tri_ET4_LT2th], Scope38/1  "PSO"
  Step10/1 -> ETM3/1(In1)  "ref_ZV"
  Constant2/1 -> Mux6/2
  ADRC 7/1(u) -> Scope36/1, enhanced5/1(Fx), [U_dk_ET4_LT2th]  "ADRC"
  enhanced5/4(the2) -> Gain9/1
  Mux6/1 -> m=5; m1=2_LT-chi bo 2/1(Input)
  enhanced5/3(the1) -> Gain10/1
  m=5; m1=2_LT-chi bo 2/1(Output) -> Demux3/1
  Demux3/3 -> PSO-ETM3/4(Input2)
  Gain9/1 -> [Teta2_ET4_LT2th], Scope33/1
  [Teta1_ET4_LT2th] -> Mux/5  "PSO_2th"
  [Teta2_ET4_LT2th] -> Mux1/5  "PSO_2th"
  [Vi_tri_ET4_LT2th] -> Mux2/5  "PSO_2th"
  [U_dk_ET4_LT2th] -> Mux3/5  "PSO_2th"
  [L_ET4] -> Mux7/2  "ET4"
  [L_nIS] -> Mux7/1  "nIS"
  [L_ET4_LT2th] -> Mux7/5  "PSO_2th"
  [L_ET4_LT] -> Mux7/4  "PSO_LT"
  Mux7/1 -> L/1
  [L_ET4_PSO] -> Mux7/3  "PSO"
  enhanced6/3(the1) -> Gain11/1
  enhanced6/1(x) -> ADRC 9/2(x), [Vi_tri_ET4_LT2], Scope46/1  "PSO"
  ADRC 9/1(u) -> Scope44/1, [U_dk_ET4_LT2], enhanced6/1(Fx)  "ADRC"
  Gain12/1 -> [Teta2_ET4_LT2], Scope41/1
  m=5; m1=2_LT-bo 1/1(Output) -> Demux4/1
  ADRC 12/1(u) -> enhanced6/2(Fl), Scope45/1  "ADRC"
  Demux4/3 -> Display15/1, PSO-ETM5/4(Input2)
  PSO-ETM6/1(ref) -> ADRC 9/1(ref), Scope43/1  "ref_ZV"
  enhanced6/4(the2) -> Gain12/1
  Step12/1 -> PSO-ETM5/1(In1)  "ref_ZV"
  Demux5/2 -> PSO-ETM6/3(Input1)
  Demux4/2 -> Display14/1, PSO-ETM5/3(Input1)
  Constant3/1 -> Mux8/2
  Gain11/1 -> [Teta1_ET4_LT2], Scope40/1
  Demux5/3 -> PSO-ETM6/4(Input2)
  enhanced6/2(l) -> Scope47/1, [L_ET4_LT2], ADRC 12/2(x), Mux8/1  "Length"
  m=5; m1=2_LT-bo 2/1(Output) -> Demux5/1
  PSO-ETM5/1(Out1) -> PSO-ETM6/1(In1), Scope42/1  "ref_ZV"
  Demux4/1 -> PSO-ETM5/2(Input), Display13/1
  Mux8/1 -> m=5; m1=2_LT-bo 2/1(Input), m=5; m1=2_LT-bo 1/1(Input)
  Demux5/1 -> PSO-ETM6/2(Input)
  Step13/1 -> ADRC 12/1(ref)  "ref_ZV"
  [Teta1_ET4_LT2] -> Mux/6  "PSO_LT2"
  [Teta2_ET4_LT2] -> Mux1/6  "PSO_LT2"
  [L_ET4_LT2] -> Mux7/6  "PSO_LT2"
  [U_dk_ET4_LT2] -> Mux3/6  "PSO_LT2"
  [Vi_tri_ET4_LT2] -> Mux2/6  "PSO_LT2"
  [x_ref] -> Mux2/7  "REF"
  [L_ref] -> Mux7/7  "REF"

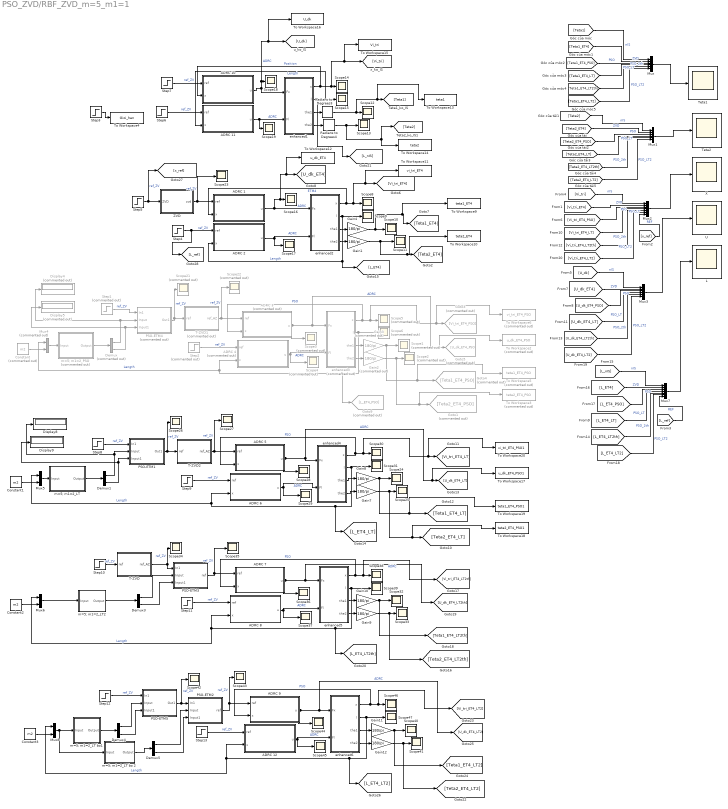
== system PSO_ZVD/RBF_ZVD_m=5_m1=1 ==
  ADRC 1 : Subsystem
  ADRC 10 : Subsystem
  ADRC 11 : Subsystem
  ADRC 12 : Subsystem
  ADRC 2 : Subsystem
  ADRC 3 : Subsystem  Commented=on
  ADRC 4 : Subsystem  Commented=on
  ADRC 5 : Subsystem
  ADRC 6 : Subsystem
  ADRC 7 : Subsystem
  ADRC 8 : Subsystem
  ADRC 9 : Subsystem
  Constant : Constant  Commented=on  Value=m2
  Constant1 : Constant  Value=m2
  Constant2 : Constant  Value=m2
  Constant3 : Constant  Value=m2
  Demux : Demux  Commented=on  Outputs=2
  Demux{1,3..5} (4 alike) : Demux  Outputs=2
  Display4 : Display  Commented=on
  Display5 : Display  Commented=on
  Display8 : Display
  Display9 : Display
  Gain{1,4,7..12} (8 alike) : Gain  Gain=180/pi
  Gain2 : Gain  Commented=on  Gain=180/pi
  Gain3 : Gain  Commented=on  Gain=180/pi
  Goto1 : Goto  Commented=on  GotoTag=Teta2_ET4_PSO
  Goto3 : Goto  Commented=on  GotoTag=Vi_tri_ET4_PSO
  Goto4 : Goto  Commented=on  GotoTag=Teta1_ET4_PSO
  Goto5 : Goto  Commented=on  GotoTag=U_dk_ET4_PSO
  Goto9 : Goto  Commented=on  GotoTag=L_ET4_PSO
  L : Scope
  Mux : Mux  Inputs=6
  Mux1 : Mux  Inputs=6
  Mux2 : Mux  Inputs=7
  Mux3 : Mux  Inputs=6
  Mux4 : Mux  Commented=on  Inputs=2
  Mux5 : Mux  Inputs=2
  Mux6 : Mux  Inputs=2
  Mux7 : Mux  Inputs=7
  Mux8 : Mux  Inputs=2
  PSO-ETM1 : Subsystem
  PSO-ETM2 : Subsystem
  PSO-ETM3 : Subsystem
  PSO-ETM4 : Subsystem  Commented=on
  PSO-ETM5 : Subsystem
  Radians to Degrees3 : simulink_extras/Transformations/Radians to Degrees
  Radians to Degrees4 : simulink_extras/Transformations/Radians to Degrees
  Scope{1..6,21..22} (8 alike) : Scope  Commented=on
  Scope{8..19,23..47} (37 alike) : Scope
  Step1 : Step  Commented=on  Time=0  After=x_ref  SampleTime=0
  Step{5,7..8,10,12} (5 alike) : Step  Time=0  After=x_ref  SampleTime=0
  Step{4,6,9,11,13} (5 alike) : Step  Time=0  Before=l_ini  After=l_ref  SampleTime=0
  Step2 : Step  Commented=on  Time=0  Before=l_ini  After=l_ref  SampleTime=0
  Step3 : Step  Time=0  After=10  SampleTime=0
  T-ZVD : Subsystem
  T-ZVD1 : Subsystem  Commented=on
  T-ZVD2 : Subsystem
  Teta1 : Scope
  Teta2 : Scope
  To Workspace10 : ToWorkspace  VariableName=teta2_ET4  SaveFormat=Timeseries  SampleTime=-1
  To Workspace11 : ToWorkspace  VariableName=vi_tri_ET4  SaveFormat=Timeseries  SampleTime=-1
  To Workspace12 : ToWorkspace  VariableName=u_dk_ET4  SaveFormat=Timeseries  SampleTime=-1
  To Workspace13 : ToWorkspace  VariableName=teta1  SaveFormat=Timeseries  SampleTime=-1
  To Workspace14 : ToWorkspace  VariableName=teta2  SaveFormat=Timeseries  SampleTime=-1
  To Workspace15 : ToWorkspace  VariableName=Vi_tri  SaveFormat=Timeseries  SampleTime=-1
  To Workspace16 : ToWorkspace  VariableName=U_dk  SaveFormat=Timeseries  SampleTime=-1
  To Workspace17 : ToWorkspace  VariableName=u_dk_ET4_PSO1  SaveFormat=Timeseries  SampleTime=-1
  To Workspace18 : ToWorkspace  VariableName=teta2_ET4_PSO1  SaveFormat=Timeseries  SampleTime=-1
  To Workspace19 : ToWorkspace  VariableName=teta1_ET4_PSO1  SaveFormat=Timeseries  SampleTime=-1
  To Workspace2 : ToWorkspace  Commented=on  VariableName=u_dk_ET4_PSO  SaveFormat=Timeseries  SampleTime=-1
  To Workspace20 : ToWorkspace  VariableName=vi_tri_ET4_PSO1  SaveFormat=Timeseries  SampleTime=-1
  To Workspace3 : ToWorkspace  Commented=on  VariableName=teta2_ET4_PSO  SaveFormat=Timeseries  SampleTime=-1
  To Workspace4 : ToWorkspace  VariableName=Gioi_han  SaveFormat=Timeseries  SampleTime=-1
  To Workspace5 : ToWorkspace  Commented=on  VariableName=teta1_ET4_PSO  SaveFormat=Timeseries  SampleTime=-1
  To Workspace6 : ToWorkspace  Commented=on  VariableName=vi_tri_ET4_PSO  SaveFormat=Timeseries  SampleTime=-1
  To Workspace9 : ToWorkspace  VariableName=teta1_ET4  SaveFormat=Timeseries  SampleTime=-1
  U : Scope
  X : Scope
  ZVD : Subsystem
  enhanced1 : Subsystem
  enhanced2 : Subsystem
  enhanced3 : Subsystem  Commented=on
  enhanced4 : Subsystem
  enhanced5 : Subsystem
  enhanced6 : Subsystem
  m=5; m1=2_LT : Subsystem
      mask help: Radial Basis Network
      mask Display: e = 0.06;c1 = [120 150 230]/255;c2 = ([120 150 230]+0)/383;c3 = ([120 150 230]+128)/383;patch([0 1 1 0],[0 0 1 1],c1);patch([0 1 1 1-e 1-e 0+e],[0 0 1 1-e 0+e 0+e],c2);patch([0 0 1 1-e 0+e 0+e],[0 1 1 1-e 1-e 0+e],c3);plot([0 1 1 0 0],[0 0 1 1 0]);fprintf('NNET');port_label('input',1,' Input');port_label('output',1,'Output ');
  m=5; m1=2_LT bo 2 : Subsystem
      mask help: Radial Basis Network
      mask Display: e = 0.06;c1 = [120 150 230]/255;c2 = ([120 150 230]+0)/383;c3 = ([120 150 230]+128)/383;patch([0 1 1 0],[0 0 1 1],c1);patch([0 1 1 1-e 1-e 0+e],[0 0 1 1-e 0+e 0+e],c2);patch([0 0 1 1-e 0+e 0+e],[0 1 1 1-e 1-e 0+e],c3);plot([0 1 1 0 0],[0 0 1 1 0]);fprintf('NNET');port_label('input',1,' Input');port_label('output',1,'Output ');
  m=5; m1=2_LT bo1 : Subsystem
      mask help: Radial Basis Network
      mask Display: e = 0.06;c1 = [120 150 230]/255;c2 = ([120 150 230]+0)/383;c3 = ([120 150 230]+128)/383;patch([0 1 1 0],[0 0 1 1],c1);patch([0 1 1 1-e 1-e 0+e],[0 0 1 1-e 0+e 0+e],c2);patch([0 0 1 1-e 0+e 0+e],[0 1 1 1-e 1-e 0+e],c3);plot([0 1 1 0 0],[0 0 1 1 0]);fprintf('NNET');port_label('input',1,' Input');port_label('output',1,'Output ');
  m=5; m1=2_LT2 : Subsystem
      mask help: Radial Basis Network
      mask Display: e = 0.06;c1 = [120 150 230]/255;c2 = ([120 150 230]+0)/383;c3 = ([120 150 230]+128)/383;patch([0 1 1 0],[0 0 1 1],c1);patch([0 1 1 1-e 1-e 0+e],[0 0 1 1-e 0+e 0+e],c2);patch([0 0 1 1-e 0+e 0+e],[0 1 1 1-e 1-e 0+e],c3);plot([0 1 1 0 0],[0 0 1 1 0]);fprintf('NNET');port_label('input',1,' Input');port_label('output',1,'Output ');
  m=5; m1=2_PSO : Subsystem  Commented=on
      mask help: Radial Basis Network
      mask Display: e = 0.06;c1 = [120 150 230]/255;c2 = ([120 150 230]+0)/383;c3 = ([120 150 230]+128)/383;patch([0 1 1 0],[0 0 1 1],c1);patch([0 1 1 1-e 1-e 0+e],[0 0 1 1-e 0+e 0+e],c2);patch([0 0 1 1-e 0+e 0+e],[0 1 1 1-e 1-e 0+e],c3);plot([0 1 1 0 0],[0 0 1 1 0]);fprintf('NNET');port_label('input',1,' Input');port_label('output',1,'Output ');
  wires:
  ADRC 2/1(u) -> enhanced2/2(Fl), Scope17/1  "ADRC"
  ADRC 11/1(u) -> enhanced1/2(Fl), Scope19/1  "ADRC"
  ADRC 1/1(u) -> enhanced2/1(Fx), To Workspace12/1, [U_dk_ET4], Scope16/1  "ADRC"
  enhanced2/1(x) -> ADRC 1/2(x), To Workspace11/1, [Vi_tri_ET4], Scope8/1  "ETM4"
  enhanced1/3(the1) -> Radians to Degrees3/1
  enhanced2/2(l) -> [L_ET4], ADRC 2/2(x), Scope9/1  "Length"
  enhanced1/1(x) -> ADRC 10/2(x), To Workspace15/1, [Vi_tri], Scope14/1  "Position"
  Step6/1 -> ADRC 11/1(ref)  "ref_ZV"
  Step4/1 -> [L_ref], ADRC 2/1(ref)  "ref_ZV"
  enhanced1/2(l) -> Scope15/1, ADRC 11/2(x), [L_nIS]  "Length"
  Step7/1 -> ADRC 10/1(ref)  "ref_ZV"
  Gain4/1 -> To Workspace9/1, [Teta1_ET4], Scope10/1
  ZVD/1(zvd) -> ADRC 1/1(ref), Scope23/1  "ref_ZV"
  Step5/1 -> [x_ref], ZVD/1(ZVD)  "ref_ZV"
  ADRC 10/1(u) -> enhanced1/1(Fx), To Workspace16/1, [U_dk], Scope18/1  "ADRC"
  Radians to Degrees3/1 -> To Workspace13/1, [Teta1], Scope12/1
  enhanced1/4(the2) -> Radians to Degrees4/1
  enhanced2/3(the1) -> Gain4/1
  Gain1/1 -> To Workspace10/1, [Teta2_ET4], Scope11/1
  enhanced2/4(the2) -> Gain1/1
  Radians to Degrees4/1 -> [Teta2], To Workspace14/1, Scope13/1
  ADRC 4/1(u) -> enhanced3/2(Fl), Scope4/1  "ADRC"
  enhanced3/4(the2) -> Gain2/1
  Step1/1 -> PSO-ETM4/1(In1)  "ref_ZV"
  ADRC 3/1(u) -> Scope3/1, enhanced3/1(Fx), To Workspace2/1, Goto5/1  "ADRC"
  enhanced3/1(x) -> ADRC 3/2(x), To Workspace6/1, Goto3/1, Scope5/1  "PSO"
  enhanced3/2(l) -> Scope6/1, Goto9/1, ADRC 4/2(x), Mux4/1  "Length"
  Gain3/1 -> Goto4/1, To Workspace5/1, Scope1/1
  Step2/1 -> ADRC 4/1(ref)  "ref_ZV"
  enhanced3/3(the1) -> Gain3/1
  PSO-ETM4/1(Out1) -> Scope21/1, T-ZVD1/1(ref)  "ref_ZV"
  [Teta2] -> Mux1/1  "nIS"
  [U_dk] -> Mux3/1  "nIS"
  [U_dk_ET4] -> Mux3/2  "ZVD"
  [Vi_tri] -> Mux2/1  "nIS"
  [Teta2_ET4] -> Mux1/2  "ZVD"
  [Vi_tri_ET4] -> Mux2/2  "ZVD"
  [Teta1] -> Mux/1  "nIS"
  Mux2/1 -> X/1
  Mux/1 -> Teta1/1
  Mux1/1 -> Teta2/1
  Mux3/1 -> U/1
  [Teta1_ET4] -> Mux/2  "ZVD"
  Step3/1 -> To Workspace4/1
  Gain2/1 -> Goto1/1, To Workspace3/1, Scope2/1
  [Teta2_ET4_PSO] -> Mux1/3  "PSO"
  [Vi_tri_ET4_PSO] -> Mux2/3  "PSO"
  [Teta1_ET4_PSO] -> Mux/3  "PSO"
  [U_dk_ET4_PSO] -> Mux3/3  "PSO"
  Constant/1 -> Mux4/2
  Mux4/1 -> m=5; m1=2_PSO/1(Input)
  Demux/1 -> PSO-ETM4/2(Input), Display4/1
  Demux/2 -> Display5/1, PSO-ETM4/3(Input1)
  T-ZVD1/1(ref_AZ) -> ADRC 3/1(ref), Scope22/1  "ref_ZV"
  m=5; m1=2_PSO/1(Output) -> Demux/1
  Mux5/1 -> m=5; m1=2_LT/1(Input)
  Constant1/1 -> Mux5/2
  enhanced4/1(x) -> ADRC 5/2(x), To Workspace20/1, [Vi_tri_ET4_LT], Scope30/1  "PSO"
  Gain7/1 -> [Teta2_ET4_LT], To Workspace18/1, Scope25/1
  enhanced4/3(the1) -> Gain8/1
  Step9/1 -> ADRC 6/1(ref)  "ref_ZV"
  T-ZVD2/1(ref_AZ) -> ADRC 5/1(ref), Scope27/1  "ref_ZV"
  PSO-ETM1/1(Out1) -> T-ZVD2/1(ref), Scope26/1  "ref_ZV"
  ADRC 5/1(u) -> Scope28/1, enhanced4/1(Fx), To Workspace17/1, [U_dk_ET4_LT]  "ADRC"
  ADRC 6/1(u) -> enhanced4/2(Fl), Scope29/1  "ADRC"
  enhanced4/2(l) -> Scope31/1, [L_ET4_LT], ADRC 6/2(x), Mux5/1  "Length"
  m=5; m1=2_LT/1(Output) -> Demux1/1
  Gain8/1 -> [Teta1_ET4_LT], To Workspace19/1, Scope24/1
  enhanced4/4(the2) -> Gain7/1
  Step8/1 -> PSO-ETM1/1(In1)  "ref_ZV"
  [Teta1_ET4_LT] -> Mux/4  "PSO_LT"
  [Teta2_ET4_LT] -> Mux1/4  "PSO_LT"
  [Vi_tri_ET4_LT] -> Mux2/4  "PSO_LT"
  [U_dk_ET4_LT] -> Mux3/4  "PSO_LT"
  PSO-ETM3/1(ref) -> ADRC 7/1(ref), Scope35/1  "ref_ZV"
  Step11/1 -> ADRC 8/1(ref)  "ref_ZV"
  T-ZVD/1(ref_AZ) -> PSO-ETM3/1(In1), Scope34/1  "ref_ZV"
  enhanced5/2(l) -> Scope39/1, [L_ET4_LT2th], ADRC 8/2(x), Mux6/1  "Length"
  Gain10/1 -> [Teta1_ET4_LT2th], Scope32/1
  ADRC 8/1(u) -> enhanced5/2(Fl), Scope37/1  "ADRC"
  enhanced5/1(x) -> ADRC 7/2(x), [Vi_tri_ET4_LT2th], Scope38/1  "PSO"
  Step10/1 -> T-ZVD/1(ref)  "ref_ZV"
  Constant2/1 -> Mux6/2
  ADRC 7/1(u) -> Scope36/1, enhanced5/1(Fx), [U_dk_ET4_LT2th]  "ADRC"
  enhanced5/4(the2) -> Gain9/1
  Mux6/1 -> m=5; m1=2_LT2/1(Input)
  enhanced5/3(the1) -> Gain10/1
  m=5; m1=2_LT2/1(Output) -> Demux3/1
  Gain9/1 -> [Teta2_ET4_LT2th], Scope33/1
  [Teta1_ET4_LT2th] -> Mux/5  "PSO_2th"
  [Teta2_ET4_LT2th] -> Mux1/5  "PSO_2th"
  [Vi_tri_ET4_LT2th] -> Mux2/5  "PSO_2th"
  [U_dk_ET4_LT2th] -> Mux3/5  "PSO_2th"
  [L_ET4] -> Mux7/2  "ZVD"
  [L_nIS] -> Mux7/1  "nIS"
  [L_ET4_LT2th] -> Mux7/5  "PSO_2th"
  [L_ET4_LT] -> Mux7/4  "PSO_LT"
  Mux7/1 -> L/1
  [L_ET4_PSO] -> Mux7/3  "PSO"
  enhanced6/3(the1) -> Gain11/1
  enhanced6/1(x) -> ADRC 9/2(x), [Vi_tri_ET4_LT2], Scope46/1  "PSO"
  ADRC 9/1(u) -> Scope44/1, [U_dk_ET4_LT2], enhanced6/1(Fx)  "ADRC"
  Gain12/1 -> [Teta2_ET4_LT2], Scope41/1
  m=5; m1=2_LT bo1/1(Output) -> Demux4/1
  ADRC 12/1(u) -> enhanced6/2(Fl), Scope45/1  "ADRC"
  PSO-ETM2/1(ref) -> Scope43/1, ADRC 9/1(ref)  "ref_ZV"
  enhanced6/4(the2) -> Gain12/1
  Step12/1 -> PSO-ETM5/1(In1)  "ref_ZV"
  Constant3/1 -> Mux8/2
  Gain11/1 -> [Teta1_ET4_LT2], Scope40/1
  enhanced6/2(l) -> Scope47/1, [L_ET4_LT2], ADRC 12/2(x), Mux8/1  "Length"
  m=5; m1=2_LT bo 2/1(Output) -> Demux5/1
  PSO-ETM5/1(Out1) -> Scope42/1, PSO-ETM2/1(In1)  "ref_ZV"
  Mux8/1 -> m=5; m1=2_LT bo 2/1(Input), m=5; m1=2_LT bo1/1(Input)
  Step13/1 -> ADRC 12/1(ref)  "ref_ZV"
  [Teta1_ET4_LT2] -> Mux/6  "PSO_LT2"
  [Teta2_ET4_LT2] -> Mux1/6  "PSO_LT2"
  [L_ET4_LT2] -> Mux7/6  "PSO_LT2"
  [U_dk_ET4_LT2] -> Mux3/6  "PSO_LT2"
  [Vi_tri_ET4_LT2] -> Mux2/6  "PSO_LT2"
  [x_ref] -> Mux2/7  "REF"
  [L_ref] -> Mux7/7  "REF"
  Demux1/1 -> Display8/1, PSO-ETM1/2(Input)
  Demux1/2 -> PSO-ETM1/3(Input1), Display9/1
  Demux3/1 -> PSO-ETM3/2(Input)
  Demux3/2 -> PSO-ETM3/3(Input1)
  Demux5/1 -> PSO-ETM2/2(Input)
  Demux5/2 -> PSO-ETM2/3(Input1)
  Demux4/1 -> PSO-ETM5/2(Input)
  Demux4/2 -> PSO-ETM5/3(Input1)

== system PSO_ZVD/non linear model ==
  Constant : Constant  Value=0
  Model_Baocao : Subsystem
  Model_Baocao1 : Subsystem
  Scope{,1..16} (17 alike) : Scope
  Scope{17..20} (4 alike) : Scope  Commented=on
  Step : Step  Time=0  SampleTime=0
  Step1 : Step  Time=0  After=-1  SampleTime=0
  Step2 : Step  Time=0  SampleTime=0
  Step5 : Step  Time=0  SampleTime=0
  con lắc đôi1 : Subsystem
  con lắc đôi2 : Subsystem  Commented=on
  con lắc đôi4 : Subsystem
  enhanced : Subsystem
  wires:
  Step5/1 -> con lắc đôi2/1(ux), con lắc đôi2/2(ul), enhanced/1(Fx), con lắc đôi4/1(Fx)  "ref_x"
  Step/1 -> con lắc đôi4/2(Fl)  "ref_L"
  con lắc đôi4/1(x) -> Scope/1  "PSO"
  con lắc đôi4/2(l) -> Scope1/1  "Length"
  con lắc đôi4/3(the1) -> Scope2/1
  con lắc đôi4/4(the2) -> Scope3/1
  Step2/1 -> Model_Baocao/1(ut), Model_Baocao1/2(ut), con lắc đôi1/1(Fx)  "ref_x"
  con lắc đôi1/4(the2) -> Scope7/1
  con lắc đôi1/2(l) -> Scope5/1  "Length"
  con lắc đôi1/1(x) -> Scope4/1  "PSO"
  Step1/1 -> Model_Baocao1/3(ul), Model_Baocao/2(ul), con lắc đôi1/2(Fl)  "ref_L"
  con lắc đôi1/3(the1) -> Scope6/1
  Constant/1 -> Model_Baocao/3(Dt), Model_Baocao1/1(Dt)
  Model_Baocao/1(x) -> Scope8/1  "Position"
  Model_Baocao/2(l) -> Scope9/1  "Length"
  Model_Baocao/3(the) -> Scope10/1  "nIS"
  Model_Baocao1/1(x) -> Scope11/1  "Position"
  Model_Baocao1/2(l) -> Scope12/1  "Length"
  Model_Baocao1/3(the) -> Scope13/1  "nIS"
  enhanced/1(x) -> Scope14/1
  enhanced/2(the1) -> Scope15/1  "Length"
  enhanced/3(the2) -> Scope16/1
  con lắc đôi2/1(x) -> Scope17/1
  con lắc đôi2/2(l1) -> Scope18/1
  con lắc đôi2/3(denta1) -> Scope19/1
  con lắc đôi2/4(denta2) -> Scope20/1

== system PSO_ZVD/Hieu/ADRC  ==
  ref : Inport
  x : Inport  Port=2
  Gain : Gain  Gain=Kp
  Gain1 : Gain  Gain=Kd
  Gain2 : Gain  Gain=1/b0
  Observer : Subsystem
  Sum : Sum  Inputs=|+-
  Sum3 : Sum  Inputs=|+-
  Sum4 : Sum  Inputs=|+-
  u : Outport
  wires:
  Sum4/1 -> Gain2/1
  Sum/1 -> Gain/1
  Gain2/1 -> u/1, Observer/1(u)
  x/1 -> Observer/2(x)
  Sum3/1 -> Sum4/1
  Observer/2(x2) -> Gain1/1
  Gain1/1 -> Sum3/2
  Gain/1 -> Sum3/1
  ref/1 -> Sum/1
  Observer/1(x3) -> Sum4/2
  Observer/3(x1) -> Sum/2

== system PSO_ZVD/Hieu/ADRC 1 ==
  ref : Inport
  x : Inport  Port=2
  Gain : Gain  Gain=Kp1
  Gain1 : Gain  Gain=Kd1
  Gain2 : Gain  Gain=1/b1
  Observer : Subsystem
  Sum : Sum  Inputs=|+-
  Sum3 : Sum  Inputs=|+-
  Sum4 : Sum  Inputs=|+-
  u : Outport
  wires:
  Sum4/1 -> Gain2/1
  Sum/1 -> Gain/1
  Gain2/1 -> u/1, Observer/1(u)
  x/1 -> Observer/2(x)
  Sum3/1 -> Sum4/1
  Observer/2(x2) -> Gain1/1
  Gain1/1 -> Sum3/2
  Gain/1 -> Sum3/1
  ref/1 -> Sum/1
  Observer/1(x3) -> Sum4/2
  Observer/3(x1) -> Sum/2

== system PSO_ZVD/Hieu/ADRC 4 ==
  ref : Inport
  x : Inport  Port=2
  Gain : Gain  Gain=Kp
  Gain1 : Gain  Gain=Kd
  Gain2 : Gain  Gain=1/b0
  Observer : Subsystem
  Sum : Sum  Inputs=|+-
  Sum3 : Sum  Inputs=|+-
  Sum4 : Sum  Inputs=|+-
  u : Outport
  wires:
  Sum4/1 -> Gain2/1
  Sum/1 -> Gain/1
  Gain2/1 -> u/1, Observer/1(u)
  x/1 -> Observer/2(x)
  Sum3/1 -> Sum4/1
  Observer/2(x2) -> Gain1/1
  Gain1/1 -> Sum3/2
  Gain/1 -> Sum3/1
  ref/1 -> Sum/1
  Observer/1(x3) -> Sum4/2
  Observer/3(x1) -> Sum/2

== system PSO_ZVD/Hieu/ADRC 5 ==
  ref : Inport
  x : Inport  Port=2
  Gain : Gain  Gain=Kp1
  Gain1 : Gain  Gain=Kd1
  Gain2 : Gain  Gain=1/b1
  Observer : Subsystem
  Sum : Sum  Inputs=|+-
  Sum3 : Sum  Inputs=|+-
  Sum4 : Sum  Inputs=|+-
  u : Outport
  wires:
  Sum4/1 -> Gain2/1
  Sum/1 -> Gain/1
  Gain2/1 -> u/1, Observer/1(u)
  x/1 -> Observer/2(x)
  Sum3/1 -> Sum4/1
  Observer/2(x2) -> Gain1/1
  Gain1/1 -> Sum3/2
  Gain/1 -> Sum3/1
  ref/1 -> Sum/1
  Observer/1(x3) -> Sum4/2
  Observer/3(x1) -> Sum/2

== system PSO_ZVD/Hieu/ADRC 8 ==
  ref : Inport
  x : Inport  Port=2
  Gain : Gain  Gain=Kp
  Gain1 : Gain  Gain=Kd
  Gain2 : Gain  Gain=1/b0
  Observer : Subsystem
  Sum : Sum  Inputs=|+-
  Sum3 : Sum  Inputs=|+-
  Sum4 : Sum  Inputs=|+-
  u : Outport
  wires:
  Sum4/1 -> Gain2/1
  Sum/1 -> Gain/1
  Gain2/1 -> u/1, Observer/1(u)
  x/1 -> Observer/2(x)
  Sum3/1 -> Sum4/1
  Observer/2(x2) -> Gain1/1
  Gain1/1 -> Sum3/2
  Gain/1 -> Sum3/1
  ref/1 -> Sum/1
  Observer/1(x3) -> Sum4/2
  Observer/3(x1) -> Sum/2

== system PSO_ZVD/Hieu/ADRC 9 ==
  ref : Inport
  x : Inport  Port=2
  Gain : Gain  Gain=Kp1
  Gain1 : Gain  Gain=Kd1
  Gain2 : Gain  Gain=1/b1
  Observer : Subsystem
  Sum : Sum  Inputs=|+-
  Sum3 : Sum  Inputs=|+-
  Sum4 : Sum  Inputs=|+-
  u : Outport
  wires:
  Sum4/1 -> Gain2/1
  Sum/1 -> Gain/1
  Gain2/1 -> u/1, Observer/1(u)
  x/1 -> Observer/2(x)
  Sum3/1 -> Sum4/1
  Observer/2(x2) -> Gain1/1
  Gain1/1 -> Sum3/2
  Gain/1 -> Sum3/1
  ref/1 -> Sum/1
  Observer/1(x3) -> Sum4/2
  Observer/3(x1) -> Sum/2

== system PSO_ZVD/Hieu/Fitness APS ZVD ==
  e : Inport
  Abs : Abs
  Abs1 : Abs
  Integrator : Integrator
  MinMax Running Resettable : simulink/Math Operations/MinMax Running Resettable  Function=max  vinit=0.0
  Step : Step  Time=0.000001  Before=1  After=0  SampleTime=0
  IAE : Outport
  MAx : Outport  Port=2
  wires:
  Abs/1 -> Integrator/1
  Abs1/1 -> MinMax Running Resettable/1
  Step/1 -> MinMax Running Resettable/2
  e/1 -> Abs/1, Abs1/1
  Integrator/1 -> IAE/1
  MinMax Running Resettable/1 -> MAx/1

== system PSO_ZVD/Hieu/Model_1 ==
  ut : Inport
  ul : Inport  Port=2
  Dt : Inport  Port=3
  Add : Sum
  Constant : Constant  Value=-mc*g
  Constant1 : Constant  Value=mc
  Crane : MATLAB Function  TreatAsAtomicUnit=on
  Integrator{,1,3..5} (5 alike) : Integrator
  Integrator2 : Integrator  InitialCondition=l
  x : Outport
  l : Outport  Port=2
  the : Outport  Port=3
  wires:
  Integrator5/1 -> [x6]
  Integrator2/1 -> l/1, [x3]
  [x4] -> Crane/3(x4)
  Crane/1(dx1) -> Integrator/1
  Integrator1/1 -> [x2]
  [x2] -> Crane/1(x2)
  Integrator4/1 -> the/1, [x5]
  [x3] -> Crane/2(x3)
  [x6] -> Crane/5(x6)
  [x5] -> Crane/4(x5)
  Integrator/1 -> x/1, [x1]
  Integrator3/1 -> [x4]
  Crane/2(dx2) -> Integrator1/1
  ut/1 -> Crane/6(ut)
  ul/1 -> Add/2
  Constant/1 -> Add/1
  Add/1 -> Crane/7(ul)
  Crane/3(dx3) -> Integrator2/1
  Crane/4(dx4) -> Integrator3/1
  Crane/5(dx5) -> Integrator4/1
  Crane/6(dx6) -> Integrator5/1
  Dt/1 -> Crane/8(Dt)
  Constant1/1 -> Crane/9(mc)

== system PSO_ZVD/Hieu/Model_2 ==
  ut : Inport
  ul : Inport  Port=2
  Dt : Inport  Port=3
  Add : Sum
  Constant : Constant  Value=-mc*g
  Constant1 : Constant  Value=mc
  Crane : MATLAB Function  TreatAsAtomicUnit=on
  Integrator{,1,3..5} (5 alike) : Integrator
  Integrator2 : Integrator  InitialCondition=l
  x : Outport
  l : Outport  Port=2
  the : Outport  Port=3
  wires:
  Integrator5/1 -> [x6]
  Integrator2/1 -> l/1, [x3]
  [x4] -> Crane/3(x4)
  Crane/1(dx1) -> Integrator/1
  Integrator1/1 -> [x2]
  [x2] -> Crane/1(x2)
  Integrator4/1 -> the/1, [x5]
  [x3] -> Crane/2(x3)
  [x6] -> Crane/5(x6)
  [x5] -> Crane/4(x5)
  Integrator/1 -> x/1, [x1]
  Integrator3/1 -> [x4]
  Crane/2(dx2) -> Integrator1/1
  ut/1 -> Crane/6(ut)
  ul/1 -> Add/2
  Constant/1 -> Add/1
  Add/1 -> Crane/7(ul)
  Crane/3(dx3) -> Integrator2/1
  Crane/4(dx4) -> Integrator3/1
  Crane/5(dx5) -> Integrator4/1
  Crane/6(dx6) -> Integrator5/1
  Dt/1 -> Crane/8(Dt)
  Constant1/1 -> Crane/9(mc)
